simulink model "expert_simu_v2"  (R2023a)
settings: Solver=VariableStepAuto  StartTime=0.0  StopTime=200  RelTol=1e-3
values from neighbouring files (symbols this model uses):
  A1 = 0.0154    [expert_pid_script.m]    (also in optimizer.m; parametros.m; variables.mat)
  A2 = 5e-5    (= 5e-05)    [expert_pid_script.m]    (also in optimizer.m; parametros.m; variables.mat)
  az = 1    [expert_pid_script.m]    (also in optimizer.m; parametros.m = 0.5; variables.mat = 0.5)
  g = 9.8    [expert_pid_script.m]    (also in optimizer.m; parametros.m; variables.mat)
  H_star = H_max/2    (= 0.31)    [expert_pid_script.m]    (also in optimizer.m; parametros.m; variables.mat)
  Q_star = ro*A2*az*sqrt(2*g*H_star)    [expert_pid_script.m]    (also in optimizer.m; parametros.m; variables.mat = 0.0616238590158)
  Qmax = 0.5    [expert_pid_script.m]    (also in optimizer.m; parametros.m; variables.mat)
  ro = 1000    [expert_pid_script.m]    (also in optimizer.m; parametros.m; variables.mat)
  st = 0.001    [parametros.m]    (also in variables.mat)
libraries: simulink x3
settings Model: Creator=empg0  LastModifiedBy=empg0
settings DebuggingCC: AlgebraicLoopMsg=none

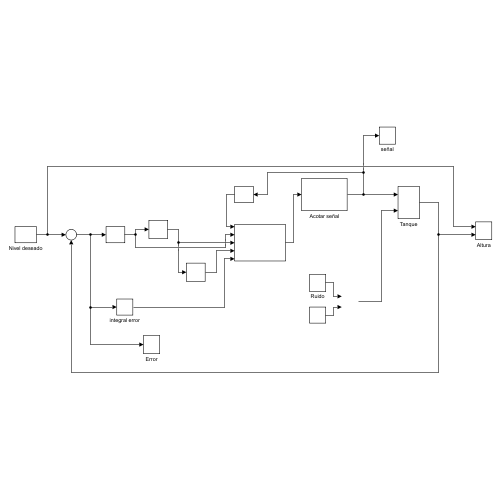
[thumbnail: Simulink's stored preview of the top-level diagram]
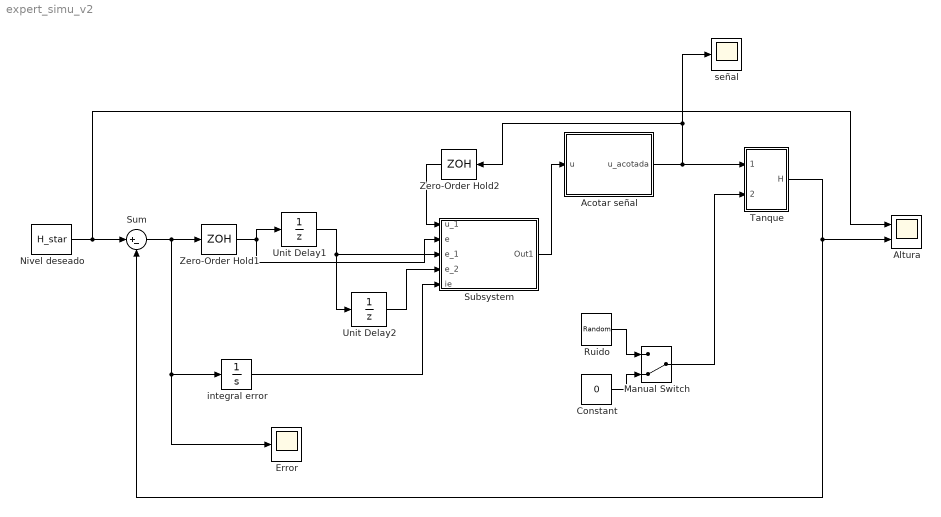
== system expert_simu_v2 ==
  Acotar señal : Subsystem
  Altura : Scope  NumInputPorts=2
  Constant : Constant  Value=0
  Error : Scope
  Manual Switch : ManualSwitch  CurrentSetting=0
  Nivel deseado : Constant  Value=H_star
  Ruido : UniformRandomNumber  Minimum=-Q_star*0.3  Maximum=Q_star*0.3  Seed=140  SampleTime=0.5
  Subsystem : Subsystem
  Sum : Sum  Inputs=|+-
  Tanque : Subsystem
  Unit Delay1 : UnitDelay  SampleTime=st  HasFrameUpgradeWarning=on
  Unit Delay2 : UnitDelay  SampleTime=st  HasFrameUpgradeWarning=on
  Zero-Order Hold1 : ZeroOrderHold  SampleTime=st
  Zero-Order Hold2 : ZeroOrderHold  SampleTime=st
  integral error : Integrator
  señal : Scope
  wires:
  Tanque/1(H) -> Sum/2, Altura/2
  Manual Switch/1 -> Tanque/2(Ruido)
  Nivel deseado/1 -> Altura/1, Sum/1
  Ruido/1 -> Manual Switch/1
  Constant/1 -> Manual Switch/2
  Sum/1 -> Zero-Order Hold1/1, Error/1, integral error/1
  Zero-Order Hold1/1 -> Unit Delay1/1, Subsystem/2(e)
  Unit Delay1/1 -> Subsystem/3(e_1), Unit Delay2/1
  Acotar señal/1(u_acotada) -> señal/1, Zero-Order Hold2/1, Tanque/1(Flujo)
  Zero-Order Hold2/1 -> Subsystem/1(u_1)
  Unit Delay2/1 -> Subsystem/4(e_2)
  integral error/1 -> Subsystem/5(ie)
  Subsystem/1(Out1) -> Acotar señal/1(u)

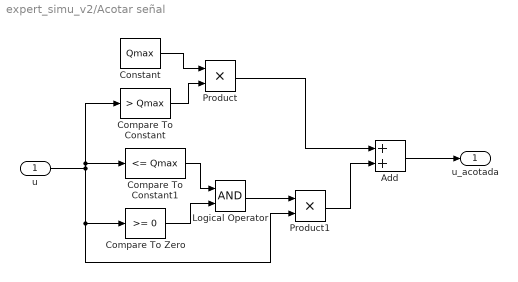
== system expert_simu_v2/Acotar señal ==
  u : Inport
  Add : Sum
  Compare To Constant : simulink/Logic and Bit Operations/Compare To Constant  relop=>  const=Qmax  OutDataTypeStr=boolean
  Compare To Constant1 : simulink/Logic and Bit Operations/Compare To Constant  relop=<=  const=Qmax  OutDataTypeStr=boolean
  Compare To Zero : simulink/Logic and Bit Operations/Compare To Zero  relop=>=  OutDataTypeStr=boolean
  Constant : Constant  Value=Qmax
  Logical Operator : Logic  AllPortsSameDT=off  OutDataTypeStr=boolean
  Product : Product
  Product1 : Product
  u_acotada : Outport
  wires:
  u/1 -> Product1/2, Compare To Zero/1, Compare To Constant1/1, Compare To Constant/1
  Compare To Constant/1 -> Product/2
  Constant/1 -> Product/1
  Compare To Constant1/1 -> Logical Operator/1
  Compare To Zero/1 -> Logical Operator/2
  Logical Operator/1 -> Product1/1
  Add/1 -> u_acotada/1
  Product1/1 -> Add/2
  Product/1 -> Add/1

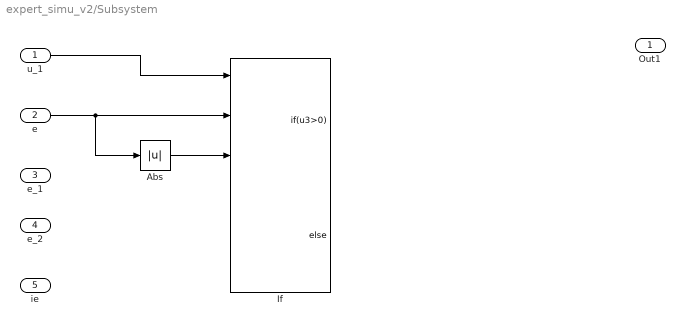
== system expert_simu_v2/Subsystem ==
  u_1 : Inport
  e : Inport  Port=2
  e_1 : Inport  Port=3
  e_2 : Inport  Port=4
  ie : Inport  Port=5
  Abs : Abs  SaturateOnIntegerOverflow=off
  If : If  NumInputs=6  IfExpression=u3>0
  Out1 : Outport
  wires:
  e/1 -> If/2, Abs/1
  Abs/1 -> If/3
  u_1/1 -> If/1

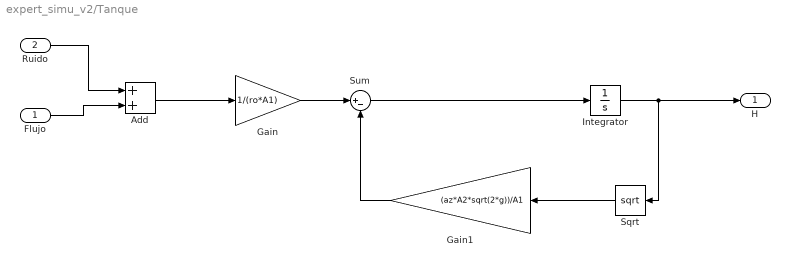
== system expert_simu_v2/Tanque ==
  Flujo : Inport
  Ruido : Inport  Port=2
  Add : Sum
  Gain : Gain  Gain=1/(ro*A1)
  Gain1 : Gain  Gain=(az*A2*sqrt(2*g))/A1
  Integrator : Integrator  LimitOutput=on  UpperSaturationLimit=0.62  LowerSaturationLimit=0
  Sqrt : Sqrt
  Sum : Sum  Inputs=|+-
  H : Outport
  wires:
  Gain/1 -> Sum/1
  Sum/1 -> Integrator/1
  Sqrt/1 -> Gain1/1
  Gain1/1 -> Sum/2
  Integrator/1 -> H/1, Sqrt/1
  Add/1 -> Gain/1
  Flujo/1 -> Add/2
  Ruido/1 -> Add/1
